simulink model "sourceTCP"  (R2021b)
settings: Solver=FixedStepAuto  StartTime=0.0  StopTime=10.0  RelTol=1e-3
libraries: simulink x1, instrumentlib x1
settings Model: DataDictionary=theSystem.sldd  Creator=samwarner  LastModifiedBy=samwarner
settings SolverCC: ConcurrentTasks=on  ZeroCrossControl=DisableAll
settings DataIOCC: SaveOutput=off  SaveTime=off
settings GRTTargetCC: CombineOutputUpdateFcns=off  MatFileLogging=off

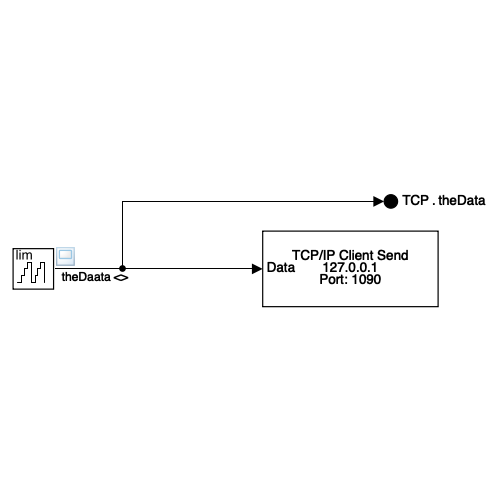
[thumbnail: Simulink's stored preview of the top-level diagram]
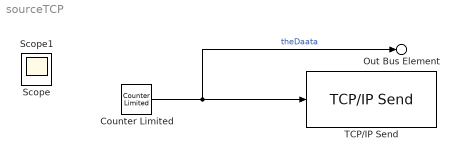
== system sourceTCP ==
  Counter Limited : simulink/Sources/Counter Limited  uplimit=3  tsamp=1
  TCP/IP Send : instrumentlib/TCP//IP Send  Host=127.0.0.1  Port=1090  ByteOrder=little-endian  EnableBlockingMode=off  Timeout=10  TransferDelay=off  SimulateUsing=Interpreted execution
  Out Bus Element : Outport  PortName=TCP  Element=theData
  Scope : Scope
  Scope1 : Scope
  wires:
  Counter Limited/1 -> TCP/IP Send/1, Out Bus Element/1  "theDaata"
